simulink model "trilink_rmic"  (R2020a)
settings: Solver=ode4  StartTime=0.0  StopTime=15  FixedStep=params.sample_time  RelTol=1e-3  EnableMultiTasking=on
settings Model: Creator=Lars  LastModifiedBy=User
settings DataIOCC: LimitDataPoints=on  SaveFormat=Array  ReturnWorkspaceOutputs=off
settings OptimizationCC: LifeSpan=inf
settings DebuggingCC: UnderspecifiedInitializationDetection=Classic  MergeDetectMultiDrivingBlocksExec=none  SolverPrmCheckMsg=warning  AllowSymbolicDim=off  SFUnexpectedBacktrackingDiag=warning  SFNoUnconditionalDefaultTransitionDiag=warning  SFExecutionAtInitializationDiag=none  ArithmeticOperatorsInVariantConditions=warning
settings HardwareCC: ProdBitPerPointer=32  ProdBitPerSizeT=32  ProdBitPerPtrDiffT=32  ProdLargestAtomicFloat=None  ProdIntDivRoundTo=Undefined  ProdEndianess=Unspecified  ProdWordSize=32  ProdHWDeviceType=32-bit Generic
settings ModelReferenceCC: PropagateSignalLabelsOutOfModel=off
settings SFSimCC: SimUseLocalCustomCode=off  CustomCodeUndefinedFunction=UseInterfaceOnly
settings RTWCC: RTWUseLocalCustomCode=off
settings CodeAppCC: StateflowObjectComments=on
settings GRTTargetCC: TargetLangStandard=C89/C90 (ANSI)
settings ConfigComp: CovMetricSettings=dw  CovHtmlReporting=on  CovSaveCumulativeToWorkspaceVar=on  CovSaveSingleToWorkspaceVar=on  CovExternalEMLEnable=off

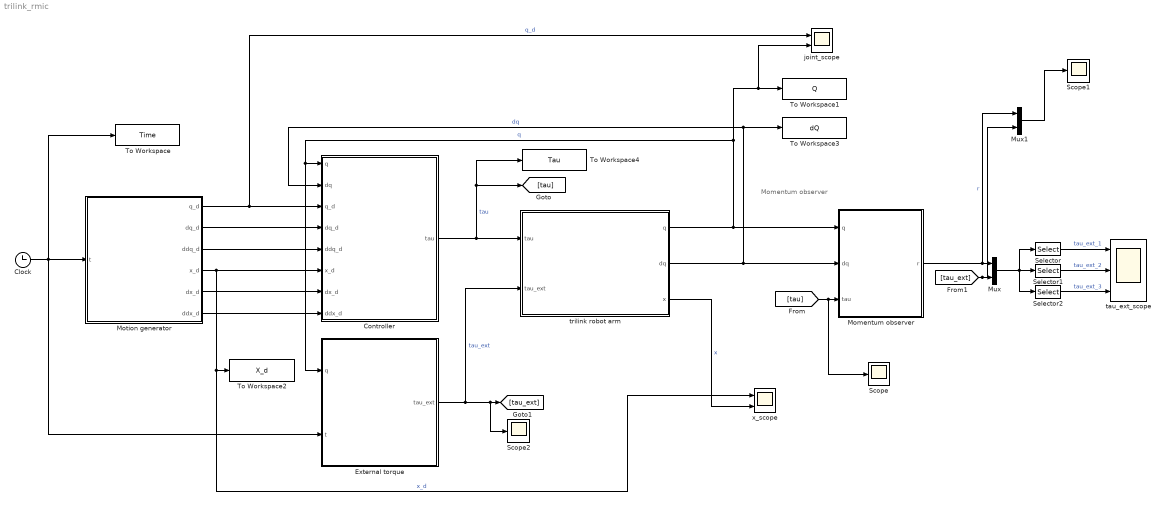
== system trilink_rmic ==
  note: Momentum observer
  Clock : Clock
  Controller : MATLAB Function  TreatAsAtomicUnit=on
  External torque : MATLAB Function  TreatAsAtomicUnit=on
  Momentum observer : Subsystem
  Motion generator : MATLAB Function  TreatAsAtomicUnit=on
  Mux : Mux  Inputs=2
  Mux1 : Mux  Inputs=2
  Scope : Scope
  Scope1 : Scope
  Scope2 : Scope
  Selector : Selector  InputPortWidth=6  IndexOptions=Index vector (dialog)  Indices=[1 4]  OutputSizes=1
  Selector1 : Selector  InputPortWidth=6  IndexOptions=Index vector (dialog)  Indices=[2 5]  OutputSizes=1
  Selector2 : Selector  InputPortWidth=6  IndexOptions=Index vector (dialog)  Indices=[3 6]  OutputSizes=1
  To Workspace : ToWorkspace  VariableName=Time  SampleTime=-1
      settings: Save2DSignal=2-D array (concatenate along first dimension)
  To Workspace1 : ToWorkspace  VariableName=Q  SampleTime=-1
      settings: Save2DSignal=2-D array (concatenate along first dimension)
  To Workspace2 : ToWorkspace  VariableName=X_d  SampleTime=-1
      settings: Save2DSignal=2-D array (concatenate along first dimension)
  To Workspace3 : ToWorkspace  VariableName=dQ  SampleTime=-1
      settings: Save2DSignal=2-D array (concatenate along first dimension)
  To Workspace4 : ToWorkspace  VariableName=Tau  SampleTime=-1
      settings: Save2DSignal=2-D array (concatenate along first dimension)
  joint_scope : Scope  NumInputPorts=2
  tau_ext_scope : Scope  NumInputPorts=3
  trilink robot arm : Subsystem
      mask Display:
      | %image(imread('/home/fernando/LRZ Sync+Share/repositories/rmic/sose_2021/additional_material/planar_arm_simplified.png'))
      | % ud = get_param(gcb,'UserData');
      | % image(ud.x)
      | image(imread('./planar_3dof.png'))
      | 
      | port_label('input', 1, '\tau','interpreter','tex')
      | port_label('input', 2, '\tau_{ext}','interpreter','tex')
      | 
      | port_label('output', 1, 'q','interpreter','tex')
      | port_label('output', 2, 'dq','interpreter','tex')
      | port_label('output', 3, 'x','interpreter','tex')
  x_scope : Scope  NumInputPorts=2
  wires:
  trilink robot arm/2("dq ") -> Momentum observer/2(dq), Controller/2(dq), To Workspace3/1  "dq"
  Clock/1 -> External torque/2(t), To Workspace/1, Motion generator/1(t)
  Motion generator/6(ddx_d) -> Controller/8(ddx_d)
  Motion generator/5(dx_d) -> Controller/7(dx_d)
  Motion generator/4(x_d) -> x_scope/1, To Workspace2/1, Controller/6(x_d)  "x_d"
  Motion generator/3(ddq_d) -> Controller/5(ddq_d)
  Motion generator/2(dq_d) -> Controller/4(dq_d)
  Motion generator/1(q_d) -> joint_scope/1, Controller/3(q_d)  "q_d"
  External torque/1(tau_ext) -> Scope2/1, [tau_ext], trilink robot arm/2(tau_ext)  "tau_ext"
  Controller/1(tau) -> To Workspace4/1, [tau], trilink robot arm/1(tau)  "tau"
  trilink robot arm/1("q ") -> Momentum observer/1(q), joint_scope/2, To Workspace1/1, External torque/1(q), Controller/1(q)  "q"
  Selector/1 -> tau_ext_scope/1  "tau_ext_1"
  Selector1/1 -> tau_ext_scope/2  "tau_ext_2"
  Selector2/1 -> tau_ext_scope/3  "tau_ext_3"
  Mux/1 -> Selector/1, Selector2/1, Selector1/1
  trilink robot arm/3(x) -> x_scope/2  "x"
  Momentum observer/1(r) -> Mux1/1, Mux/1  "r"
  [tau] -> Scope/1, Momentum observer/3(tau)
  [tau_ext] -> Mux1/2, Mux/2
  Mux1/1 -> Scope1/1

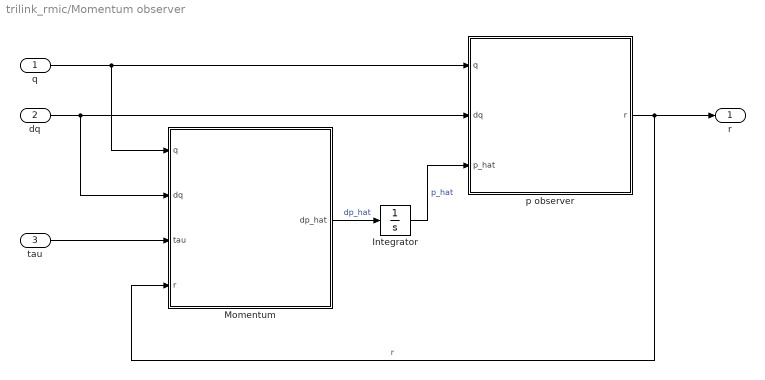
== system trilink_rmic/Momentum observer ==
  q : Inport
  dq : Inport  Port=2
  tau : Inport  Port=3
  Integrator : Integrator  InitialCondition=zeros(3,1)
  Momentum : MATLAB Function  TreatAsAtomicUnit=on
  p observer : MATLAB Function  TreatAsAtomicUnit=on
  r : Outport
  wires:
  p observer/1(r) -> Momentum/4(r), r/1  "r"
  Momentum/1(dp_hat) -> Integrator/1  "dp_hat"
  Integrator/1 -> p observer/3(p_hat)  "p_hat"
  tau/1 -> Momentum/3(tau)
  q/1 -> p observer/1(q), Momentum/1(q)
  dq/1 -> Momentum/2(dq), p observer/2(dq)

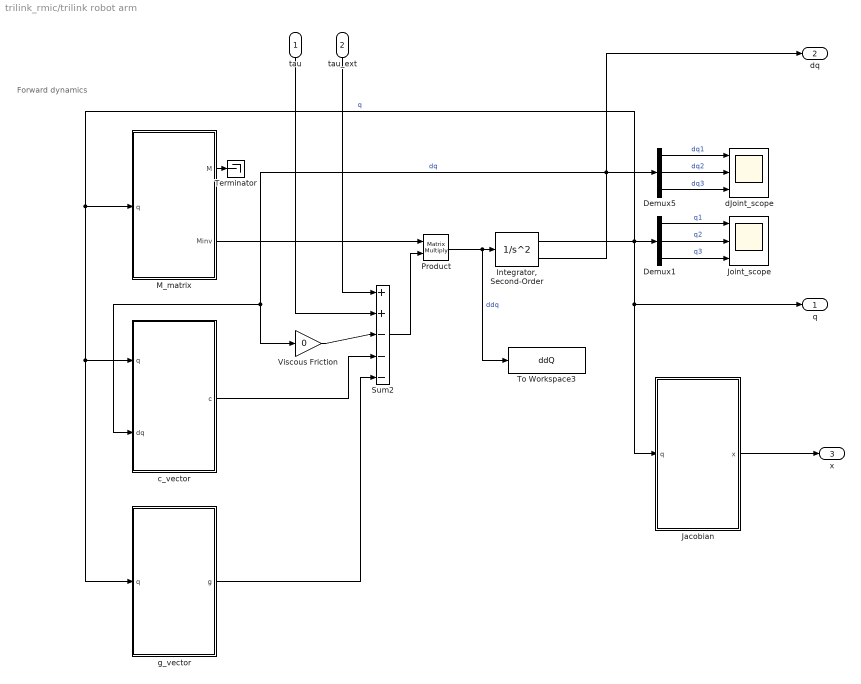
== system trilink_rmic/trilink robot arm ==
  note: Forward dynamics
  tau : Inport
  tau_ext : Inport  Port=2
  Demux1 : Demux  Outputs=3
  Demux5 : Demux  Outputs=3
  "Integrator, Second-Order" : SecondOrderIntegrator  ICX=params.q0  ICDXDT=params.dq0
  Jacobian : MATLAB Function  TreatAsAtomicUnit=on
  Joint_scope : Scope  NumInputPorts=3
  M_matrix : MATLAB Function  TreatAsAtomicUnit=on
  Product : Product  Multiplication=Matrix(*)
  Sum2 : Sum  Inputs=++|---
  Terminator : Terminator
  To Workspace3 : ToWorkspace  VariableName=ddQ  SampleTime=-1
      settings: Save2DSignal=2-D array (concatenate along first dimension)
  Viscous Friction : Gain  Gain=0
  c_vector : MATLAB Function  TreatAsAtomicUnit=on
  dJoint_scope : Scope  NumInputPorts=3
  g_vector : MATLAB Function  TreatAsAtomicUnit=on
  "q " : Outport
  "dq " : Outport  Port=2
  x : Outport  Port=3
  wires:
  Demux1/1 -> Joint_scope/1  "q1"
  Demux1/2 -> Joint_scope/2  "q2"
  "Integrator, Second-Order"/2 -> c_vector/2(dq), Viscous Friction/1, "dq "/1, Demux5/1  "dq"
  Demux5/1 -> dJoint_scope/1  "dq1"
  "Integrator, Second-Order"/1 -> Demux1/1, Jacobian/1(q), "q "/1, g_vector/1(q), c_vector/1(q), M_matrix/1(q)  "q"
  M_matrix/2(Minv) -> Product/1
  Demux5/2 -> dJoint_scope/2  "dq2"
  Sum2/1 -> Product/2
  M_matrix/1(M) -> Terminator/1
  Product/1 -> To Workspace3/1, "Integrator, Second-Order"/1  "ddq"
  g_vector/1(g) -> Sum2/5
  c_vector/1(c) -> Sum2/4
  Viscous Friction/1 -> Sum2/3
  tau/1 -> Sum2/2
  tau_ext/1 -> Sum2/1
  Demux5/3 -> dJoint_scope/3  "dq3"
  Demux1/3 -> Joint_scope/3  "q3"
  Jacobian/1(x) -> x/1

== matlab function trilink_rmic/trilink robot arm/Jacobian ==
  data: q input; x output; params parameter
function x = fkinematics(q, params)
%     J  = planar3R_Jac(q,params);
    x    = planar3R_fkin(q,params);
end

== matlab function trilink_rmic/External torque ==
  data: q input; t input; tau_ext output; params parameter
function tau_ext = exernal_torque(q, t, params)
    tau_ext = calc_tau_ext(q, params, t);
end

== matlab function trilink_rmic/Controller ==
  data: q input; dq input; q_d input; dq_d input; ddq_d input; x_d input; dx_d input; ddx_d input; tau output; params parameter
function tau = controller(q, dq, q_d, dq_d, ddq_d, x_d, dx_d, ddx_d, params)
    t  = 0;
    switch params.controller
        case 0
            % PD controller
            tau = ctrl_PD(t,q,q_d,dq,dq_d);
        case 1
            % Impedance controller (redundant, translation only)
            tau = ctrl_imp_R(t,q,dq,x_d,dx_d,ddx_d,params);
        case 2
            % Impedance controller (x,y,phi)
            tau = ctrl_imp(t,q,dq,x_d,dx_d,ddx_d,params);
        otherwise
            % No torques if no controller is selected
            tau = zeros(length(params.pkin),1);
    end
end

== matlab function trilink_rmic/Momentum observer/Momentum ==
  data: q input; dq input; tau input; r input; dp_hat output; params parameter
function dp_hat = momentum_estimate(q, dq, tau, r, params)
    dp_hat = calc_dp_hat(q, dq, tau, r, params);
end

== matlab function trilink_rmic/trilink robot arm/c_vector ==
  data: q input; dq input; c output; params parameter
function c = c_vector(q, dq, params)
    if params.flag_reg
        c = planar3R_C_reg(q, dq, params)*dq;
    else
        c = planar3R_c(q, dq, params.pkin(1:2), params.m, params.rSges, params.Icges);
    end

== matlab function trilink_rmic/trilink robot arm/g_vector ==
  data: g output; q input; params parameter
function g = g_vector(q, params)
    if params.flag_reg
        g = planar3R_g_reg(q, params);
    else
        g = planar3R_g(q, params.g_base, params.pkin(1:2), params.m, params.rSges);
    end

== matlab function trilink_rmic/trilink robot arm/M_matrix ==
  data: M output; q input; params parameter; Minv output
function [M, Minv] = M_matrix(q, params)
    if params.flag_reg
        M    = planar3R_M_reg(q,params);
    else
        M    = planar3R_M(q,params.pkin(1:2), params.m, params.rSges, params.Icges);
    end
    Minv = pinv(M);

== matlab function trilink_rmic/Motion generator ==
  data: t input; q_d output; dq_d output; ddq_d output; x_d output; dx_d output; ddx_d output; params parameter
function [q_d, dq_d, ddq_d, x_d, dx_d, ddx_d] = desired_trajectory(t, params)
    [q_d, dq_d, ddq_d, x_d, dx_d, ddx_d] = motion_generator(t, params);
end

== matlab function trilink_rmic/Momentum observer/p observer ==
  data: q input; dq input; p_hat input; r output; params parameter
function r = residual(q,dq, p_hat, params)
    r = p_observer(q,dq, p_hat, params);
end
